simulink model "PI"  (R2024b)
settings: Solver=VariableStepAuto  StartTime=0.0  StopTime=10.0  RelTol=1e-3
settings Model: Creator=Ilya  LastModifiedBy=Ilya

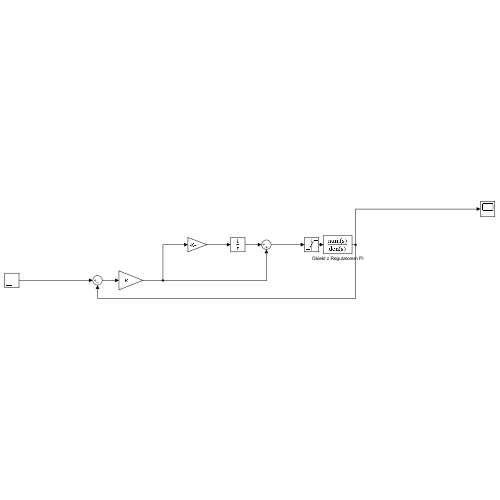
[thumbnail: Simulink's stored preview of the top-level diagram]
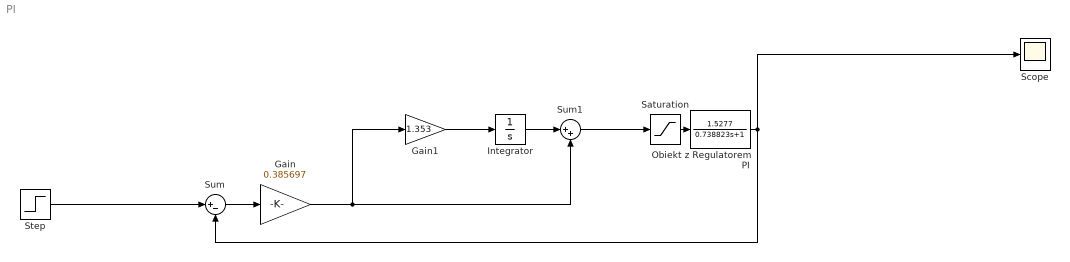
== system PI ==
  Gain : Gain  Gain=0.385697
  Gain1 : Gain  Gain=1.353
  Integrator : Integrator
  Obiekt z Regulatorem PI : TransferFcn  Numerator=[1.5277]  Denominator=[0.738823 1]
  Saturation : Saturate  UpperLimit=1000  LowerLimit=0
  Scope : Scope
  Step : Step  Time=0  After=100  SampleTime=0
  Sum : Sum  Inputs=|+-
  Sum1 : Sum  Inputs=|++
  wires:
  Sum1/1 -> Saturation/1
  Step/1 -> Sum/1
  Gain1/1 -> Integrator/1
  Obiekt z Regulatorem PI/1 -> Scope/1, Sum/2
  Gain/1 -> Gain1/1, Sum1/2
  Integrator/1 -> Sum1/1
  Saturation/1 -> Obiekt z Regulatorem PI/1
  Sum/1 -> Gain/1
